simulink model "jellystone_v5"  (R2016b)
settings: Solver=FixedStepAuto  StartTime=0.0  StopTime=30  FixedStep=1  RelTol=1e-3
values from neighbouring files (symbols this model uses):
  C0 = 2.017+(rand-.5)*.404    [executeModel.m]    (also in project.m)
  E0 = 31.217+(rand-.5)*6.244    [executeModel.m]    (also in project.m)
  G0 = .8+(rand-.5)*.16    [executeModel.m]    (also in project.m)
  W0 = 0    [executeModel.m]    (also in project.m)
settings Model: Creator=thomaskennedy  LastModifiedBy=thomaskennedy
settings DebuggingCC: InitInArrayFormatMsg=none

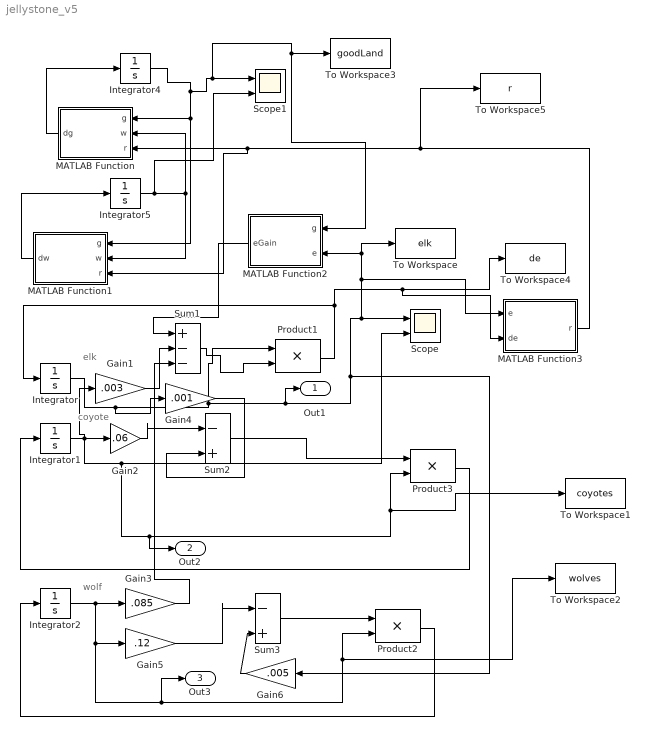
== system jellystone_v5 ==
  note: elk
  note: coyote
  note: wolf
  Gain1 : Gain  Gain=.003  SaturateOnIntegerOverflow=on  OutDataTypeStr=Inherit: Same as input  ParamDataTypeStr=Inherit: Same as input
  Gain2 : Gain  Gain=.06  SaturateOnIntegerOverflow=on  OutDataTypeStr=Inherit: Same as input  ParamDataTypeStr=Inherit: Same as input
  Gain3 : Gain  Gain=.085  SaturateOnIntegerOverflow=on  OutDataTypeStr=Inherit: Same as input  ParamDataTypeStr=Inherit: Same as input
  Gain4 : Gain  Gain=.001  SaturateOnIntegerOverflow=on  OutDataTypeStr=Inherit: Same as input  ParamDataTypeStr=Inherit: Same as input
  Gain5 : Gain  Gain=.12  SaturateOnIntegerOverflow=on  OutDataTypeStr=Inherit: Same as input  ParamDataTypeStr=Inherit: Same as input
  Gain6 : Gain  Gain=.005  SaturateOnIntegerOverflow=on  OutDataTypeStr=Inherit: Same as input  ParamDataTypeStr=Inherit: Same as input
  Integrator : Integrator  InitialCondition=E0
  Integrator1 : Integrator  InitialCondition=C0
  Integrator2 : Integrator  InitialCondition=W0
  Integrator4 : Integrator  InitialCondition=G0
  Integrator5 : Integrator  InitialCondition=1-G0
  MATLAB Function : MATLAB Function  TreatAsAtomicUnit=on
  MATLAB Function1 : MATLAB Function  TreatAsAtomicUnit=on
  MATLAB Function2 : MATLAB Function  TreatAsAtomicUnit=on
  MATLAB Function3 : MATLAB Function  TreatAsAtomicUnit=on
  Product1 : Product  SaturateOnIntegerOverflow=on  InputSameDT=on  OutDataTypeStr=Inherit: Same as first input
  Product2 : Product  SaturateOnIntegerOverflow=on  InputSameDT=on  OutDataTypeStr=Inherit: Same as first input
  Product3 : Product  SaturateOnIntegerOverflow=on  InputSameDT=on  OutDataTypeStr=Inherit: Same as first input
  Scope : Scope  NumInputPorts=2
  Scope1 : Scope  NumInputPorts=2
  Sum1 : Sum  Inputs=|+||-||-|  SaturateOnIntegerOverflow=on  InputSameDT=on  OutDataTypeStr=Inherit: Same as first input
  Sum2 : Sum  Inputs=|-||+|  SaturateOnIntegerOverflow=on  InputSameDT=on  OutDataTypeStr=Inherit: Same as first input
  Sum3 : Sum  Inputs=|-||+|  SaturateOnIntegerOverflow=on  InputSameDT=on  OutDataTypeStr=Inherit: Same as first input
  To Workspace : ToWorkspace  VariableName=elk  SampleTime=-1
  To Workspace1 : ToWorkspace  VariableName=coyotes  SampleTime=-1
  To Workspace2 : ToWorkspace  VariableName=wolves  SampleTime=-1
  To Workspace3 : ToWorkspace  VariableName=goodLand  SampleTime=-1
  To Workspace4 : ToWorkspace  VariableName=de  SampleTime=-1
  To Workspace5 : ToWorkspace  VariableName=r  SampleTime=-1
  Out1 : Outport
  Out2 : Outport  Port=2
  Out3 : Outport  Port=3
  wires:
  MATLAB Function2/1(eGain) -> Sum1/1
  Integrator1/1 -> Gain2/1, Out2/1, To Workspace1/1, Product3/2, Scope/2, Gain1/1
  Integrator/1 -> Gain4/1, Out1/1, Gain6/1, Scope/1, MATLAB Function3/1(e), MATLAB Function2/2(e), To Workspace/1, Product1/1
  Product1/1 -> MATLAB Function3/2(de), To Workspace4/1, Integrator/1
  Sum2/1 -> Product3/1
  Product3/1 -> Integrator1/1
  Sum1/1 -> Product1/2
  Gain1/1 -> Sum1/2
  Integrator2/1 -> Out3/1, To Workspace2/1, Product2/2, Gain5/1, Gain3/1
  Gain3/1 -> Sum1/3
  Gain2/1 -> Sum2/1
  Gain4/1 -> Sum2/2
  Gain5/1 -> Sum3/1
  Gain6/1 -> Sum3/2
  Sum3/1 -> Product2/1
  Product2/1 -> Integrator2/1
  Integrator4/1 -> MATLAB Function2/1(g), To Workspace3/1, Scope1/1, MATLAB Function1/1(g), MATLAB Function/1(g)
  Integrator5/1 -> Scope1/2, MATLAB Function1/2(w), MATLAB Function/2(w)
  MATLAB Function1/1(dw) -> Integrator5/1
  MATLAB Function/1(dg) -> Integrator4/1
  MATLAB Function3/1(r) -> To Workspace5/1, MATLAB Function1/3(r), MATLAB Function/3(r)

== matlab function jellystone_v5/MATLAB Function1 ==
  data: g input; dw output; w input; r input
function dw = fcn(g,w,r)

dw = .4*w*(1-w-1.07*g*(.31*r+g)/(r+g));

== matlab function jellystone_v5/MATLAB Function ==
  data: g input; dg output; w input; r input
function dg = fcn(g,w,r)
dg=.27*g*(1-g-.6*w*(r+g)/(.31*r+g));

== matlab function jellystone_v5/MATLAB Function2 ==
  data: g input; eGain output; e input
function eGain = fcn(g,e)

if(g*40>e)
    eGain = .04;
else
    eGain =0;
end

== matlab function jellystone_v5/MATLAB Function3 ==
  data: e input; de input; r output
function r = fcn(e,de)

r = e/(e+de)-1;
